simulink model "Flowchart1"  (Simulink 6.0)
settings: Solver=FixedStepDiscrete  StartTime=0.0  StopTime=10.0  RelTol=1e-3
settings Model: Creator=scaife  LastModifiedBy=scaife  ExtModeAutoUpdateStatusClock=off

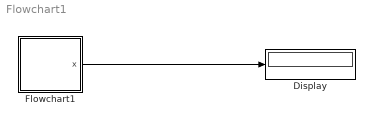
== system Flowchart1 ==
  Display : Display
  Flowchart1 : Stateflow chart
  wires:
  Flowchart1/1(x) -> Display/1

== stateflow chart Flowchart1 ==
  state A [parallel]
    (default) -> (junction 4) : {x++;}
  data: x output int32
